simulink model "OMSblk_bw"  (Simulink 7.0)
settings: Solver=ode45  SolverMode=SingleTasking  StartTime=0.0  StopTime=999999  MaxStep=10  RelTol=1e-3  AbsTol=1e-3
undefined symbols (not defined in the file): k, TI
settings Model: Creator=lfd  LastModifiedBy=lfd  ExtModeAutoUpdateStatusClock=off
settings DataIOCC: LimitDataPoints=off  SaveOutput=off  SaveTime=off
settings OptimizationCC: BlockReduction=off  BooleanDataType=off
settings DebuggingCC: SaveWithParameterizedLinksMsg=none  SignalResolutionControl=TryResolveAllWithWarning  SolverPrmCheckMsg=none  MultiTaskDSMMsg=warning  MultiTaskCondExecSysMsg=none  StrictBusMsg=None
settings HardwareCC: TargetUnknown=on
settings RTWCC: IncludeERTFirstTime=on
settings GRTTargetCC: TargetFcnLib=ansi_tfl_tmw.mat  ModelReferenceCompliant=off  MatFileLogging=off

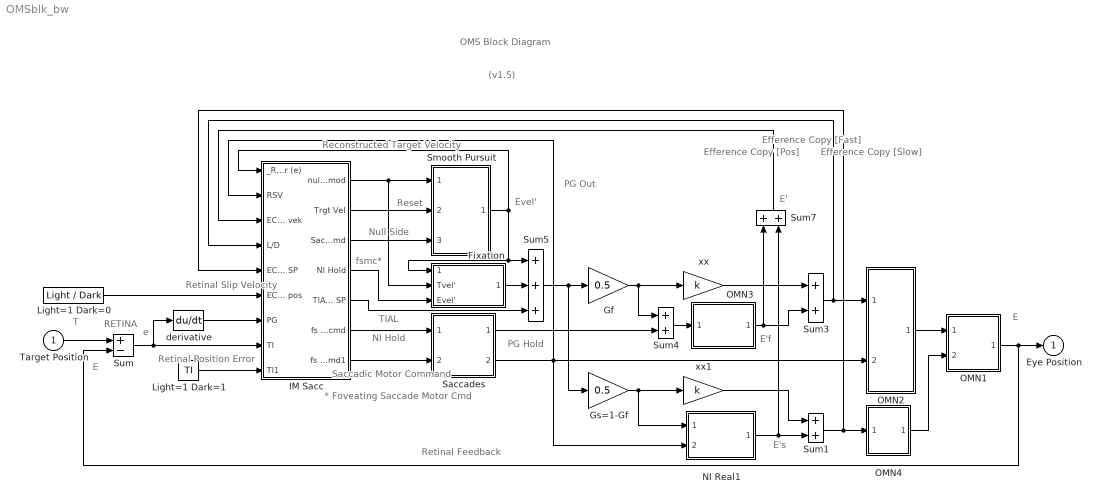
== system OMSblk_bw ==
  note: OMS Block Diagram
  note: PG Hold
  note: Saccadic Motor
      | Command
  note: Reconstructed
      | Target  Velocity
  note: Efference
      | Copy
      | [Pos]
  note: Efference
      | Copy
      | [Fast]
  note: Retinal Position Error
  note: E
  note: e
  note: E
  note: T
  note: Retinal Feedback
  note: Evel'
  note: E'f
  note: Retinal Slip
      | Velocity
  note: RETINA
  note: fsmc*
  note: * Foveating Saccade Motor Cmd
  note: Null Side
  note: (v1.5)
  note: TIAL
  note: NI Hold
  note: Reset
  note: Efference
      | Copy
      | [Slow]
  note: PG Out
  note: E's
  note: E'
  Target Position : Inport  OutDataType=sfix(16)  OutScaling=2^0
  Fixation : Subsystem
      mask Display: disp('Fixation')
  Gf : Gain  Gain=0.5  ParameterDataType=sfix(16)  ParameterScaling=2^0  OutDataType=sfix(16)  OutScaling=2^0  SaturateOnIntegerOverflow=on
  Gs=1-Gf : Gain  Gain=0.5  ParameterDataType=sfix(16)  ParameterScaling=2^0  OutDataType=sfix(16)  OutScaling=2^0  SaturateOnIntegerOverflow=on
  IM Sacc : Subsystem
      mask Display: disp('INTERNAL\nMONITOR\n[Sacc,FS/BS,\nSP,AL,\nNI Control]')
  Light=1 Dark=0 : Constant  Value=Light / Dark  OutDataType=sfix(16)  OutScaling=2^0
  Light=1 Dark=1 : Constant  Value=TI  OutDataType=sfix(16)  OutScaling=2^0
  NI Real1 : Subsystem
      mask Display: disp('rNeural\nIntegrator\n(Slow)')
  OMN1 : Subsystem
      mask Display: disp('OM\nPlant')
  OMN2 : Subsystem
      mask Display: disp('OMN\n(Fast)\n[Tonic +\nPhasic]')
  OMN3 : Subsystem
      mask Display: disp('Neural \nIntegrator\n(Fast)')
  OMN4 : Subsystem
      mask Display: disp('OMN\n(Slow)\n[Tonic]')
  Saccades : Subsystem
      mask Display: disp('Saccadic\n[PG,rNI\nNI Hold]')
  Smooth Pursuit : Subsystem
      mask Display: disp('Smooth\nPursuit')
  Sum : Sum  Inputs=+-  OutDataType=sfix(16)  OutScaling=2^0  SaturateOnIntegerOverflow=on  InputSameDT=on
  Sum1 : Sum  OutDataType=sfix(16)  OutScaling=2^0  SaturateOnIntegerOverflow=on  InputSameDT=on
  Sum3 : Sum  OutDataType=sfix(16)  OutScaling=2^0  SaturateOnIntegerOverflow=on  InputSameDT=on
  Sum4 : Sum  OutDataType=sfix(16)  OutScaling=2^0  SaturateOnIntegerOverflow=on  InputSameDT=on
  Sum5 : Sum  Inputs=+++  OutDataType=sfix(16)  OutScaling=2^0  SaturateOnIntegerOverflow=on  InputSameDT=on
  Sum7 : Sum  Orientation=up  OutDataType=sfix(16)  OutScaling=2^0  SaturateOnIntegerOverflow=on  InputSameDT=on
  derivative : Derivative
      mask Display: disp('s')
  xx : Gain  Gain=k  ParameterDataType=sfix(16)  ParameterScaling=2^0  OutDataType=sfix(16)  OutScaling=2^0  SaturateOnIntegerOverflow=on
  xx1 : Gain  Gain=k  ParameterDataType=sfix(16)  ParameterScaling=2^0  OutDataType=sfix(16)  OutScaling=2^0  SaturateOnIntegerOverflow=on
  Eye Position : Outport  OutDataType=sfix(16)  OutScaling=2^0  InitialOutput=0
  wires:
  xx/1 -> Sum3/1
  OMN3/1(out_1) -> Sum3/2, Sum7/1
  Sum3/1 -> OMN2/1(from NI), IM Sacc/4(L/D)
  OMN2/1(out_1) -> OMN1/1(from NI)
  OMN1/1(out_1) -> Eye Position/1, Sum/2
  Sum4/1 -> OMN3/1(from NI)
  Sum5/1 -> Gf/1, Gs=1-Gf/1
  Target Position/1 -> Sum/1
  xx1/1 -> Sum1/1
  NI Real1/1(NIOUT [epospr]) -> Sum1/2, Sum7/2
  Sum1/1 -> IM Sacc/5(ECPY P + SP), OMN4/1(from NI)
  OMN4/1(out_1) -> OMN1/2(from PG)
  derivative/1 -> IM Sacc/7(PG)
  Sum/1 -> IM Sacc/8(TI), derivative/1
  Light=1 Dark=1/1 -> IM Sacc/9(TI1)
  IM Sacc/1(null mod) -> Smooth Pursuit/1(trgt pos), Fixation/2(Tvel')
  IM Sacc/2(Trgt Vel) -> Smooth Pursuit/2(null mod)
  IM Sacc/3(Sacc Mot Cmd) -> Smooth Pursuit/3(null mod1)
  IM Sacc/7(fs mot cmd1) -> Saccades/2()
  IM Sacc/6(fs mot cmd) -> Saccades/1(trgt pos)
  IM Sacc/5(TIAL + SP) -> Sum5/3
  Fixation/1(" CorrVel [velcorr]") -> Sum5/2
  Smooth Pursuit/1(eye pos) -> Sum5/1, Fixation/1(fs [fsmc30]), IM Sacc/1(_RetErr (e))
  IM Sacc/4(NI Hold) -> Fixation/3(Evel')
  Sum7/1 -> IM Sacc/3(ECPY vek)
  Light=1 Dark=0/1 -> IM Sacc/6(ECPY pos)
  Saccades/2(eye pos1) -> OMN2/2(from PG), IM Sacc/2(RSV), NI Real1/2(PG + (TIAL+SP)1)
  Saccades/1(eye pos) -> Sum4/2
  Gf/1 -> xx/1, Sum4/1
  Gs=1-Gf/1 -> xx1/1, NI Real1/1(PG + (TIAL+SP))

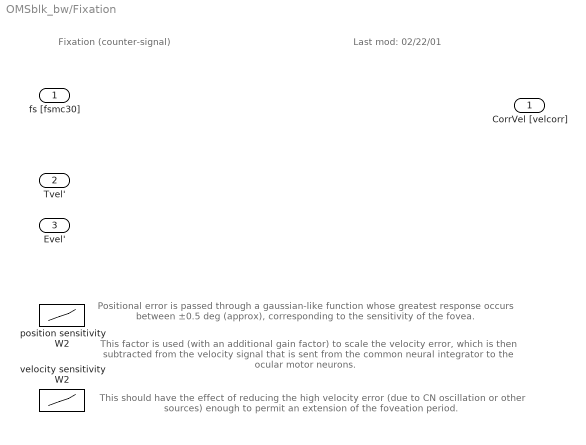
== system OMSblk_bw/Fixation ==
  note: Fixation (counter-signal)
  note: Last mod: 02/22/01
  note: Positional error is passed through a gaussian-like function whose greatest
      | response occurs between ±0.5 deg (approx), corresponding to the sensitivity
      | of the fovea.
  note: This factor is used (with an additional gain factor) to scale the velocity error,
      | which is then subtracted from the velocity signal that is sent from the
      | common neural integrator to the ocular motor neurons.
  note: This should have the effect of reducing the high velocity error (due
      | to CN oscillation or other sources) enough to permit an extension of
      | the foveation period.
  fs [fsmc30] : Inport  OutDataType=sfix(16)  OutScaling=2^0
  Tvel' : Inport  Port=2  OutDataType=sfix(16)  OutScaling=2^0
  Evel' : Inport  Port=3  OutDataType=sfix(16)  OutScaling=2^0
  position sensitivity W2 : Lookup  InputValues="[-5 -2  -1 -0.5   0.5   1    2    5]"  Table="[ 0   0.125    0.5     1      1     0.5    0.125  0]"  OutDataType=sfix(16)  OutScaling=2^0  SaturateOnIntegerOverflow=on
  velocity sensitivity W2 : Lookup  InputValues="[-30 -15   -8  -4   4     8  15  30]"  Table="[0  0.125   0.5    1    1    0.5   0.125  0]"  OutDataType=sfix(16)  OutScaling=2^0  SaturateOnIntegerOverflow=on
  " CorrVel [velcorr]" : Outport  OutDataType=sfix(16)  OutScaling=2^0  InitialOutput=0
  wires:
  ? -> " CorrVel [velcorr]"/1

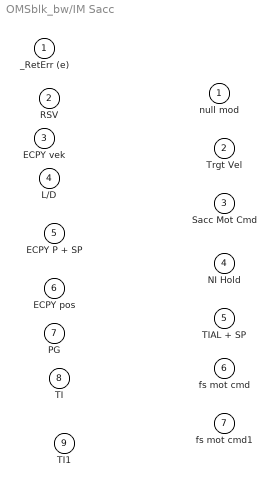
== system OMSblk_bw/IM Sacc ==
  _RetErr (e) : Inport  OutDataType=sfix(16)  OutScaling=2^0
  RSV : Inport  Port=2  OutDataType=sfix(16)  OutScaling=2^0
  ECPY vek : Inport  Port=3  OutDataType=sfix(16)  OutScaling=2^0
  L/D : Inport  Port=4  OutDataType=sfix(16)  OutScaling=2^0
  ECPY P + SP : Inport  Port=5  OutDataType=sfix(16)  OutScaling=2^0
  ECPY pos : Inport  Port=6  OutDataType=sfix(16)  OutScaling=2^0
  PG : Inport  Port=7  OutDataType=sfix(16)  OutScaling=2^0
  TI : Inport  Port=8  OutDataType=sfix(16)  OutScaling=2^0
  TI1 : Inport  Port=9  OutDataType=sfix(16)  OutScaling=2^0
  null mod : Outport  OutDataType=sfix(16)  OutScaling=2^0  InitialOutput=0
  Trgt Vel : Outport  Port=2  OutDataType=sfix(16)  OutScaling=2^0  InitialOutput=0
  Sacc Mot Cmd : Outport  Port=3  OutDataType=sfix(16)  OutScaling=2^0  InitialOutput=0
  NI Hold : Outport  Port=4  OutDataType=sfix(16)  OutScaling=2^0  InitialOutput=0
  TIAL + SP : Outport  Port=5  OutDataType=sfix(16)  OutScaling=2^0  InitialOutput=0
  fs mot cmd : Outport  Port=6  OutDataType=sfix(16)  OutScaling=2^0  InitialOutput=0
  fs mot cmd1 : Outport  Port=7  OutDataType=sfix(16)  OutScaling=2^0  InitialOutput=0

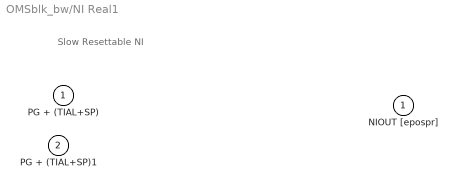
== system OMSblk_bw/NI Real1 ==
  note: Slow Resettable NI
  PG + (TIAL+SP) : Inport  OutDataType=sfix(16)  OutScaling=2^0
  PG + (TIAL+SP)1 : Inport  Port=2  OutDataType=sfix(16)  OutScaling=2^0
  NIOUT [epospr] : Outport  OutDataType=sfix(16)  OutScaling=2^0  InitialOutput=0

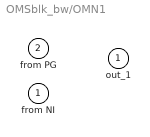
== system OMSblk_bw/OMN1 ==
  from NI : Inport  OutDataType=sfix(16)  OutScaling=2^0
  from PG : Inport  Port=2  OutDataType=sfix(16)  OutScaling=2^0
  out_1 : Outport  OutDataType=sfix(16)  OutScaling=2^0  InitialOutput=0

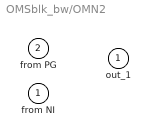
== system OMSblk_bw/OMN2 ==
  from NI : Inport  OutDataType=sfix(16)  OutScaling=2^0
  from PG : Inport  Port=2  OutDataType=sfix(16)  OutScaling=2^0
  out_1 : Outport  OutDataType=sfix(16)  OutScaling=2^0  InitialOutput=0

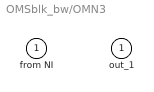
== system OMSblk_bw/OMN3 ==
  from NI : Inport  OutDataType=sfix(16)  OutScaling=2^0
  out_1 : Outport  OutDataType=sfix(16)  OutScaling=2^0  InitialOutput=0

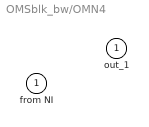
== system OMSblk_bw/OMN4 ==
  from NI : Inport  OutDataType=sfix(16)  OutScaling=2^0
  out_1 : Outport  OutDataType=sfix(16)  OutScaling=2^0  InitialOutput=0

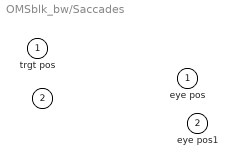
== system OMSblk_bw/Saccades ==
  trgt pos : Inport  OutDataType=sfix(16)  OutScaling=2^0
   : Inport  Port=2  OutDataType=sfix(16)  OutScaling=2^0
  eye pos : Outport  OutDataType=sfix(16)  OutScaling=2^0  InitialOutput=0
  eye pos1 : Outport  Port=2  OutDataType=sfix(16)  OutScaling=2^0  InitialOutput=0

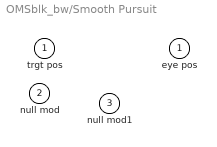
== system OMSblk_bw/Smooth Pursuit ==
  trgt pos : Inport  OutDataType=sfix(16)  OutScaling=2^0
  null mod : Inport  Port=2  OutDataType=sfix(16)  OutScaling=2^0
  null mod1 : Inport  Port=3  OutDataType=sfix(16)  OutScaling=2^0
  eye pos : Outport  OutDataType=sfix(16)  OutScaling=2^0  InitialOutput=0
